simulink model "t2a"  (R2018b)
settings: Solver=VariableStepAuto  StartTime=0.0  StopTime=10.0  RelTol=1e-3
settings Model: Creator=anton  LastModifiedBy=anton

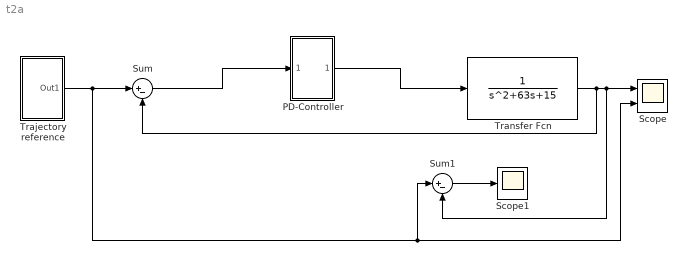
== system t2a ==
  "PD-Controller " : Subsystem
  Scope : Scope  NumInputPorts=2
  Scope1 : Scope
  Sum : Sum  Inputs=|+-
  Sum1 : Sum  Inputs=|+-
  "Trajectory reference " : Subsystem
  Transfer Fcn : TransferFcn  Denominator=[1 63 15]
  wires:
  Transfer Fcn/1 -> Scope/1, Sum1/2, Sum/2
  "Trajectory reference "/1(Out1) -> Scope/2, Sum1/1, Sum/1
  Sum1/1 -> Scope1/1
  Sum/1 -> "PD-Controller "/1(In1)
  "PD-Controller "/1(Out1) -> Transfer Fcn/1

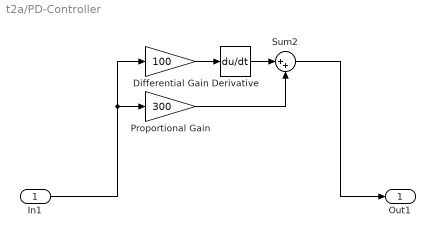
== system t2a/PD-Controller  ==
  In1 : Inport
  Derivative : Derivative
  Differential Gain : Gain  Gain=100
  "Proportional Gain " : Gain  Gain=300
  Sum2 : Sum  Inputs=|++
  Out1 : Outport
  wires:
  "Proportional Gain "/1 -> Sum2/2
  Sum2/1 -> Out1/1
  In1/1 -> "Proportional Gain "/1, Differential Gain/1
  Differential Gain/1 -> Derivative/1
  Derivative/1 -> Sum2/1

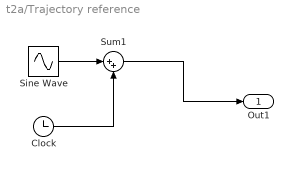
== system t2a/Trajectory reference  ==
  Clock : Clock
      settings: Decimation=20
  Sine Wave : Sin  SampleTime=0
  Sum1 : Sum  Inputs=|++
  Out1 : Outport
  wires:
  Clock/1 -> Sum1/2
  Sum1/1 -> Out1/1
  Sine Wave/1 -> Sum1/1
